simulink model "ThreePhaseBidirectional"  (R2020b)
settings: Solver=ode23t  StartTime=0.0  StopTime=0.5  RelTol=1e-3
libraries: powerlib x27, powerlib_meascontrol x6, pid_lib x4, eePowerMeasurement x4, simulink x2
settings Model: Creator=Matthew  LastModifiedBy=Matthew

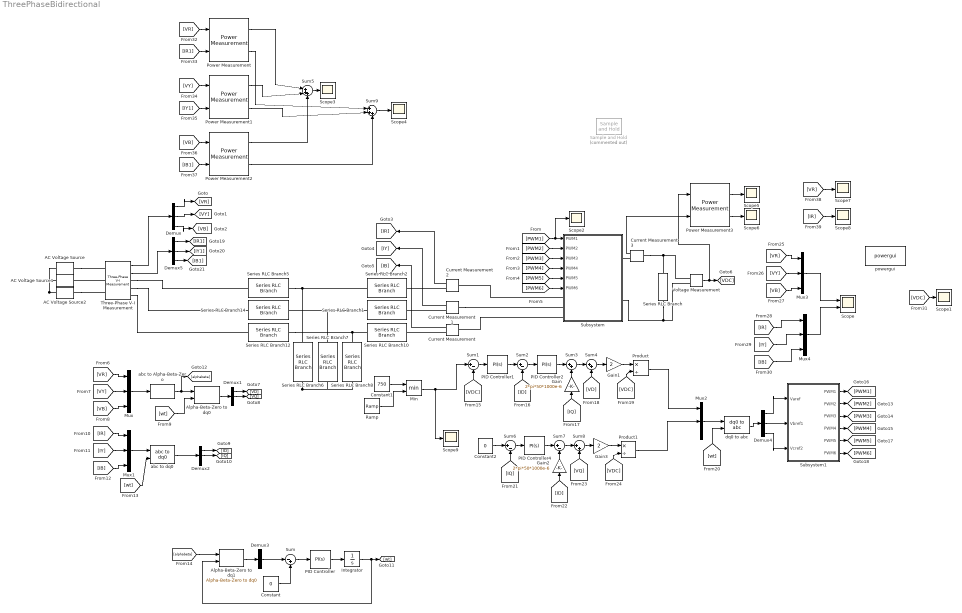
== system ThreePhaseBidirectional ==
  AC Voltage Source : powerlib/Electrical Sources/AC Voltage Source  Amplitude=350  Phase=0  Frequency=50  SampleTime=0  Measurements=None  BusType=swing  Pref=10e3  Qref=0  Qmin=-inf  Qmax=+inf
  AC Voltage Source1 : powerlib/Electrical Sources/AC Voltage Source  Amplitude=350  Phase=120  Frequency=50  SampleTime=0  Measurements=None  BusType=swing  Pref=10e3  Qref=0  Qmin=-inf  Qmax=+inf
  AC Voltage Source2 : powerlib/Electrical Sources/AC Voltage Source  Amplitude=350  Phase=240  Frequency=50  SampleTime=0  Measurements=None  BusType=swing  Pref=10e3  Qref=0  Qmin=-inf  Qmax=+inf
  Alpha-Beta-Zero to dq0 : powerlib_meascontrol/Transformations/Alpha-Beta-Zero to dq0  Alignment=90 degrees behind phase A axis
  Alpha-Beta-Zero to dq1 : powerlib_meascontrol/Transformations/Alpha-Beta-Zero to dq0  Alignment=90 degrees behind phase A axis
  Constant : Constant  Value=0
  Constant1 : Constant  Value=750
  Constant2 : Constant  Value=0
  Current Measurement{,1..3} (4 alike) : powerlib/Measurements/Current Measurement  PhasorSimulation=off  OutputType=Complex  PSBequivalent=0
  Demux{,1..5} (6 alike) : Demux  Outputs=3
  Gain : Gain  Gain=2*pi*50*1000e-6
  Gain1 : Gain  Gain=2
  Gain2 : Gain  Gain=2*pi*50*1000e-6
  Gain3 : Gain  Gain=2
  Integrator : Integrator
  Min : MinMax  Inputs=2
  Mux{,1..4} (5 alike) : Mux  Inputs=3
  PID Controller : pid_lib/PID Controller  Controller=PI  Form=Parallel  TimeDomain=Continuous-time  UseExternalTs=off  SampleTime=-1  IntegratorMethod=Forward Euler  FilterMethod=Forward Euler  ControllerParametersSource=internal  P=10  I=50000  D=0  UseFilter=on  N=100  TunerSelectOption=Transfer Function Based (PID Tuner App)  InitialConditionSource=internal  InitialConditionForIntegrator=0  InitialConditionForFilter=0  DifferentiatorICPrevScaledInput=0  ExternalReset=none  TrackingMode=off  Kt=1  LimitOutput=off  SatLimitsSource=internal  UpperSaturationLimit=inf  LowerSaturationLimit=-inf  LinearizeAsGain=on  AntiWindupMode=none  Kb=1  POutMin=[]  POutMax=[]  IOutMin=[]  IOutMax=[]  DOutMin=[]  DOutMax=[]  NOutMin=[]  NOutMax=[]  SumOutMin=[]  SumOutMax=[]  SaturationOutMin=[]  SaturationOutMax=[]  PParamMin=[]  PParamMax=[]  IParamMin=[]  IParamMax=[]  DParamMin=[]  DParamMax=[]  NParamMin=[]  NParamMax=[]  KbParamMin=[]  KbParamMax=[]  KtParamMin=[]  KtParamMax=[]  KbOutMin=[]  KbOutMax=[]  KtOutMin=[]  KtOutMax=[]  IntegratorOutMin=[]  IntegratorOutMax=[]  FilterOutMin=[]  FilterOutMax=[]  SumI1OutMin=[]  SumI1OutMax=[]  SumI2OutMin=[]  SumI2OutMax=[]  SumI3OutMin=[]  SumI3OutMax=[]  SumI4OutMin=[]  SumI4OutMax=[]  SumDOutMin=[]  SumDOutMax=[]  DifferentiatorOutMin=[]  DifferentiatorOutMax=[]  FilterDiffOutCoefMin=[]  FilterDiffOutCoefMax=[]  ReciprocalOutMin=[]  ReciprocalOutMax=[]  SumDenOutMin=[]  SumDenOutMax=[]  SumNumOutMin=[]  SumNumOutMax=[]  DivideOutMin=[]  DivideOutMax=[]  UdiffTsProdOutMin=[]  UdiffTsProdOutMax=[]  NTsProdOutMin=[]  NTsProdOutMax=[]  UintegralTsProdOutMin=[]  UintegralTsProdOutMax=[]  UngainTsProdOutMin=[]  UngainTsProdOutMax=[]  IntegratorContinuousStateAttributes=''  IntegratorStateMustResolveToSignalObject=off  IntegratorRTWStateStorageClass=Auto  FilterContinuousStateAttributes=''  FilterStateMustResolveToSignalObject=off  FilterRTWStateStorageClass=Auto  ParallelPVariant=InternalParameters  IdealPVariant=Disabled  IVariant=InternalParameters  DVariant=Disabled  IntegratorVariant=Continuous  SatVariant=Disabled  AWVariant=Passthrough  PCopyVariant=Disabled  TRVariant=Disabled  FdbkBlocksVariant=Forward  IdealPFdbkVariant=Disabled  SatFdbkVariant=Disabled  DerivativeFilterVariant=Disabled  NVariant=Disabled  NCopyVariant=Disabled_SignalSpec  FilterICVariant=Disabled  IntegratorICVariant=InternalICs  ExternalResetVariant=Disabled  TRSumVariant=Passthrough  SumFdbkVariant=Disabled  SumVariant=Sum_PI  TsampFilterVariant=InternalTs  TsampNgainVariant=Passthrough  TsampIntegralVariant=Passthrough  ExternalSaturationOutDataTypeStr=Inherit: Same as second input
  PID Controller1 : pid_lib/PID Controller  Controller=PI  Form=Parallel  TimeDomain=Continuous-time  UseExternalTs=off  SampleTime=-1  IntegratorMethod=Forward Euler  FilterMethod=Forward Euler  ControllerParametersSource=internal  P=0.5  I=200  D=0  UseFilter=on  N=100  TunerSelectOption=Transfer Function Based (PID Tuner App)  InitialConditionSource=internal  InitialConditionForIntegrator=0  InitialConditionForFilter=0  DifferentiatorICPrevScaledInput=0  ExternalReset=none  TrackingMode=off  Kt=1  LimitOutput=off  SatLimitsSource=internal  UpperSaturationLimit=inf  LowerSaturationLimit=-inf  LinearizeAsGain=on  AntiWindupMode=none  Kb=1  POutMin=[]  POutMax=[]  IOutMin=[]  IOutMax=[]  DOutMin=[]  DOutMax=[]  NOutMin=[]  NOutMax=[]  SumOutMin=[]  SumOutMax=[]  SaturationOutMin=[]  SaturationOutMax=[]  PParamMin=[]  PParamMax=[]  IParamMin=[]  IParamMax=[]  DParamMin=[]  DParamMax=[]  NParamMin=[]  NParamMax=[]  KbParamMin=[]  KbParamMax=[]  KtParamMin=[]  KtParamMax=[]  KbOutMin=[]  KbOutMax=[]  KtOutMin=[]  KtOutMax=[]  IntegratorOutMin=[]  IntegratorOutMax=[]  FilterOutMin=[]  FilterOutMax=[]  SumI1OutMin=[]  SumI1OutMax=[]  SumI2OutMin=[]  SumI2OutMax=[]  SumI3OutMin=[]  SumI3OutMax=[]  SumI4OutMin=[]  SumI4OutMax=[]  SumDOutMin=[]  SumDOutMax=[]  DifferentiatorOutMin=[]  DifferentiatorOutMax=[]  FilterDiffOutCoefMin=[]  FilterDiffOutCoefMax=[]  ReciprocalOutMin=[]  ReciprocalOutMax=[]  SumDenOutMin=[]  SumDenOutMax=[]  SumNumOutMin=[]  SumNumOutMax=[]  DivideOutMin=[]  DivideOutMax=[]  UdiffTsProdOutMin=[]  UdiffTsProdOutMax=[]  NTsProdOutMin=[]  NTsProdOutMax=[]  UintegralTsProdOutMin=[]  UintegralTsProdOutMax=[]  UngainTsProdOutMin=[]  UngainTsProdOutMax=[]  IntegratorContinuousStateAttributes=''  IntegratorStateMustResolveToSignalObject=off  IntegratorRTWStateStorageClass=Auto  FilterContinuousStateAttributes=''  FilterStateMustResolveToSignalObject=off  FilterRTWStateStorageClass=Auto  ParallelPVariant=InternalParameters  IdealPVariant=Disabled  IVariant=InternalParameters  DVariant=Disabled  IntegratorVariant=Continuous  SatVariant=Disabled  AWVariant=Passthrough  PCopyVariant=Disabled  TRVariant=Disabled  FdbkBlocksVariant=Forward  IdealPFdbkVariant=Disabled  SatFdbkVariant=Disabled  DerivativeFilterVariant=Disabled  NVariant=Disabled  NCopyVariant=Disabled_SignalSpec  FilterICVariant=Disabled  IntegratorICVariant=InternalICs  ExternalResetVariant=Disabled  TRSumVariant=Passthrough  SumFdbkVariant=Disabled  SumVariant=Sum_PI  TsampFilterVariant=InternalTs  TsampNgainVariant=Passthrough  TsampIntegralVariant=Passthrough  ExternalSaturationOutDataTypeStr=Inherit: Same as second input
  PID Controller2 : pid_lib/PID Controller  Controller=PI  Form=Parallel  TimeDomain=Continuous-time  UseExternalTs=off  SampleTime=-1  IntegratorMethod=Forward Euler  FilterMethod=Forward Euler  ControllerParametersSource=internal  P=25  I=500  D=0  UseFilter=on  N=100  TunerSelectOption=Transfer Function Based (PID Tuner App)  InitialConditionSource=internal  InitialConditionForIntegrator=0  InitialConditionForFilter=0  DifferentiatorICPrevScaledInput=0  ExternalReset=none  TrackingMode=off  Kt=1  LimitOutput=off  SatLimitsSource=internal  UpperSaturationLimit=inf  LowerSaturationLimit=-inf  LinearizeAsGain=on  AntiWindupMode=none  Kb=1  POutMin=[]  POutMax=[]  IOutMin=[]  IOutMax=[]  DOutMin=[]  DOutMax=[]  NOutMin=[]  NOutMax=[]  SumOutMin=[]  SumOutMax=[]  SaturationOutMin=[]  SaturationOutMax=[]  PParamMin=[]  PParamMax=[]  IParamMin=[]  IParamMax=[]  DParamMin=[]  DParamMax=[]  NParamMin=[]  NParamMax=[]  KbParamMin=[]  KbParamMax=[]  KtParamMin=[]  KtParamMax=[]  KbOutMin=[]  KbOutMax=[]  KtOutMin=[]  KtOutMax=[]  IntegratorOutMin=[]  IntegratorOutMax=[]  FilterOutMin=[]  FilterOutMax=[]  SumI1OutMin=[]  SumI1OutMax=[]  SumI2OutMin=[]  SumI2OutMax=[]  SumI3OutMin=[]  SumI3OutMax=[]  SumI4OutMin=[]  SumI4OutMax=[]  SumDOutMin=[]  SumDOutMax=[]  DifferentiatorOutMin=[]  DifferentiatorOutMax=[]  FilterDiffOutCoefMin=[]  FilterDiffOutCoefMax=[]  ReciprocalOutMin=[]  ReciprocalOutMax=[]  SumDenOutMin=[]  SumDenOutMax=[]  SumNumOutMin=[]  SumNumOutMax=[]  DivideOutMin=[]  DivideOutMax=[]  UdiffTsProdOutMin=[]  UdiffTsProdOutMax=[]  NTsProdOutMin=[]  NTsProdOutMax=[]  UintegralTsProdOutMin=[]  UintegralTsProdOutMax=[]  UngainTsProdOutMin=[]  UngainTsProdOutMax=[]  IntegratorContinuousStateAttributes=''  IntegratorStateMustResolveToSignalObject=off  IntegratorRTWStateStorageClass=Auto  FilterContinuousStateAttributes=''  FilterStateMustResolveToSignalObject=off  FilterRTWStateStorageClass=Auto  ParallelPVariant=InternalParameters  IdealPVariant=Disabled  IVariant=InternalParameters  DVariant=Disabled  IntegratorVariant=Continuous  SatVariant=Disabled  AWVariant=Passthrough  PCopyVariant=Disabled  TRVariant=Disabled  FdbkBlocksVariant=Forward  IdealPFdbkVariant=Disabled  SatFdbkVariant=Disabled  DerivativeFilterVariant=Disabled  NVariant=Disabled  NCopyVariant=Disabled_SignalSpec  FilterICVariant=Disabled  IntegratorICVariant=InternalICs  ExternalResetVariant=Disabled  TRSumVariant=Passthrough  SumFdbkVariant=Disabled  SumVariant=Sum_PI  TsampFilterVariant=InternalTs  TsampNgainVariant=Passthrough  TsampIntegralVariant=Passthrough  ExternalSaturationOutDataTypeStr=Inherit: Same as second input
  PID Controller4 : pid_lib/PID Controller  Controller=PI  Form=Parallel  TimeDomain=Continuous-time  UseExternalTs=off  SampleTime=-1  IntegratorMethod=Forward Euler  FilterMethod=Forward Euler  ControllerParametersSource=internal  P=25  I=500  D=0  UseFilter=on  N=100  TunerSelectOption=Transfer Function Based (PID Tuner App)  InitialConditionSource=internal  InitialConditionForIntegrator=0  InitialConditionForFilter=0  DifferentiatorICPrevScaledInput=0  ExternalReset=none  TrackingMode=off  Kt=1  LimitOutput=off  SatLimitsSource=internal  UpperSaturationLimit=inf  LowerSaturationLimit=-inf  LinearizeAsGain=on  AntiWindupMode=none  Kb=1  POutMin=[]  POutMax=[]  IOutMin=[]  IOutMax=[]  DOutMin=[]  DOutMax=[]  NOutMin=[]  NOutMax=[]  SumOutMin=[]  SumOutMax=[]  SaturationOutMin=[]  SaturationOutMax=[]  PParamMin=[]  PParamMax=[]  IParamMin=[]  IParamMax=[]  DParamMin=[]  DParamMax=[]  NParamMin=[]  NParamMax=[]  KbParamMin=[]  KbParamMax=[]  KtParamMin=[]  KtParamMax=[]  KbOutMin=[]  KbOutMax=[]  KtOutMin=[]  KtOutMax=[]  IntegratorOutMin=[]  IntegratorOutMax=[]  FilterOutMin=[]  FilterOutMax=[]  SumI1OutMin=[]  SumI1OutMax=[]  SumI2OutMin=[]  SumI2OutMax=[]  SumI3OutMin=[]  SumI3OutMax=[]  SumI4OutMin=[]  SumI4OutMax=[]  SumDOutMin=[]  SumDOutMax=[]  DifferentiatorOutMin=[]  DifferentiatorOutMax=[]  FilterDiffOutCoefMin=[]  FilterDiffOutCoefMax=[]  ReciprocalOutMin=[]  ReciprocalOutMax=[]  SumDenOutMin=[]  SumDenOutMax=[]  SumNumOutMin=[]  SumNumOutMax=[]  DivideOutMin=[]  DivideOutMax=[]  UdiffTsProdOutMin=[]  UdiffTsProdOutMax=[]  NTsProdOutMin=[]  NTsProdOutMax=[]  UintegralTsProdOutMin=[]  UintegralTsProdOutMax=[]  UngainTsProdOutMin=[]  UngainTsProdOutMax=[]  IntegratorContinuousStateAttributes=''  IntegratorStateMustResolveToSignalObject=off  IntegratorRTWStateStorageClass=Auto  FilterContinuousStateAttributes=''  FilterStateMustResolveToSignalObject=off  FilterRTWStateStorageClass=Auto  ParallelPVariant=InternalParameters  IdealPVariant=Disabled  IVariant=InternalParameters  DVariant=Disabled  IntegratorVariant=Continuous  SatVariant=Disabled  AWVariant=Passthrough  PCopyVariant=Disabled  TRVariant=Disabled  FdbkBlocksVariant=Forward  IdealPFdbkVariant=Disabled  SatFdbkVariant=Disabled  DerivativeFilterVariant=Disabled  NVariant=Disabled  NCopyVariant=Disabled_SignalSpec  FilterICVariant=Disabled  IntegratorICVariant=InternalICs  ExternalResetVariant=Disabled  TRSumVariant=Passthrough  SumFdbkVariant=Disabled  SumVariant=Sum_PI  TsampFilterVariant=InternalTs  TsampNgainVariant=Passthrough  TsampIntegralVariant=Passthrough  ExternalSaturationOutDataTypeStr=Inherit: Same as second input
  Power Measurement : eePowerMeasurement/Power Measurement  LabelModeActiveChoice=Continuous  F=50  K=[1]  Ts=0
      settings: SourceProductBaseCode=PS
  Power Measurement1 : eePowerMeasurement/Power Measurement  LabelModeActiveChoice=Continuous  F=50  K=[1]  Ts=0
      settings: SourceProductBaseCode=PS
  Power Measurement2 : eePowerMeasurement/Power Measurement  LabelModeActiveChoice=Continuous  F=50  K=[1]  Ts=0
      settings: SourceProductBaseCode=PS
  Power Measurement3 : eePowerMeasurement/Power Measurement  LabelModeActiveChoice=Continuous  F=50  K=[0 1]  Ts=0
      settings: SourceProductBaseCode=PS
  Product : Product  Inputs=*/
  Product1 : Product  Inputs=*/
  Ramp : simulink/Sources/Ramp  slope=1136  start=0  InitialOutput=608
  Sample and Hold : powerlib_meascontrol/Additional Components/Sample and Hold  Commented=on  ic=0  Ts=0
      settings: SourceProductBaseCode=PS
  Scope : Scope  NumInputPorts=2
  Scope{1..9} (9 alike) : Scope
  Series RLC Branch : powerlib/Elements/Series RLC Branch  LConnTagsString=__new0  RConnTagsString=__new0  BranchType=R  Resistance=6.4  Inductance=1e-3  SetiL0=off  InitialCurrent=0  Capacitance=1e-6  Setx0=off  InitialVoltage=0  Measurements=None
  Series RLC Branch{1..2,5,10,12,14} (6 alike) : powerlib/Elements/Series RLC Branch  LConnTagsString=__new0  RConnTagsString=__new0  BranchType=L  Resistance=1  Inductance=500e-6  SetiL0=off  InitialCurrent=0  Capacitance=0  Setx0=off  InitialVoltage=0  Measurements=None
  Series RLC Branch6 : powerlib/Elements/Series RLC Branch  LConnTagsString=__new0  RConnTagsString=__new0  BranchType=C  Resistance=1  Inductance=1e-3  SetiL0=off  InitialCurrent=0  Capacitance=100e-6  Setx0=off  InitialVoltage=0  Measurements=None
  Series RLC Branch7 : powerlib/Elements/Series RLC Branch  LConnTagsString=__new0  RConnTagsString=__new0  BranchType=C  Resistance=1  Inductance=1e-3  SetiL0=off  InitialCurrent=0  Capacitance=100e-6  Setx0=off  InitialVoltage=0  Measurements=None
  Series RLC Branch8 : powerlib/Elements/Series RLC Branch  LConnTagsString=__new0  RConnTagsString=__new0  BranchType=C  Resistance=1  Inductance=1e-3  SetiL0=off  InitialCurrent=0  Capacitance=100e-6  Setx0=off  InitialVoltage=0  Measurements=None
  Subsystem : Subsystem
  Subsystem1 : Subsystem
  Sum : Sum  Inputs=|-+
  Sum{1..2,6..7} (4 alike) : Sum  Inputs=|+-
  Sum3 : Sum  Inputs=|++
  Sum4 : Sum  Inputs=|++
  Sum5 : Sum  Inputs=|+++
  Sum8 : Sum  Inputs=|++
  Sum9 : Sum  Inputs=|+++
  Three-Phase V-I Measurement : powerlib/Measurements/Three-Phase V-I Measurement  VoltageMeasurement=phase-to-phase  SetLabelV=off  LabelV=Vabc  Vpu=off  VpuLL=off  CurrentMeasurement=yes  SetLabelI=off  LabelI=Iabc  Ipu=off  Pbase=100e6  Vbase=500e3  OutputType=Complex  PhasorSimulation=off  PSBequivalent=0
  Voltage Measurement : powerlib/Measurements/Voltage Measurement  PhasorSimulation=off  OutputType=Complex  PSBequivalent=0
  abc to Alpha-Beta-Zero : powerlib_meascontrol/Transformations/abc to Alpha-Beta-Zero
  abc to dq0 : powerlib_meascontrol/Transformations/abc to dq0  Alignment=90 degrees behind phase A axis
  dq0 to abc : powerlib_meascontrol/Transformations/dq0 to abc  Alignment=90 degrees behind phase A axis
  powergui : powerlib/powergui  Priority=1  SimulationMode=Discrete  SampleTime=1e-6  frequency=60  Iterations=50  frequencyindice=50  Pbase=100e6  ErrMax=1e-4  UnitsV=kV  UnitsW=MW  buscounter=0  FunctionMessages=off  echomessages=off  EnableUseOfTLC=off  CurrentSourceSwitches=off  DisableSnubberDevices=off  DisableRonSwitches=off  DisableVfSwitches=off  DisplayEquations=off  AutomaticDiscreteSolvers=off  SolverType=Tustin/Backward Euler (TBE)  Interpol=off  ExternalGateDelay=off  methode=off  Ts=100  x0status=blocks  SPID=on  SwTol=0  HookPort=off  NonlinearTolerance=1e-4  nMaxIteration=100  ContinueOnMaxIteration=off  RestoreLinks=warning  ResistiveCurrentMeasurement=off  Frange=[0:2:500]  Ylog=off  Xlog=on  ShowGrid=off  save=off  variable=ZData  structure=0  ZoomFFT=off  StartTime=0.0  cycles=1  DisplayStyle=1  fundamental=60  FreqAxis=off  MaxFrequency=1000  frequencyindicesteady=1  RmsSteady=1  display=off
  wires:
  Three-Phase V-I Measurement/1 -> Demux/1
  Demux/1 -> [VR]
  Demux/2 -> [VY]
  Demux/3 -> [VB]
  Current Measurement2/1 -> [IR]
  Current Measurement1/1 -> [IY]
  Current Measurement/1 -> [IB]
  [PWM1] -> Scope2/1, Subsystem/1(PWM1)
  [PWM2] -> Subsystem/2(PWM2)
  [PWM3] -> Subsystem/3(PWM3)
  [PWM4] -> Subsystem/4(PWM4)
  [PWM5] -> Subsystem/5(PWM5)
  [PWM6] -> Subsystem/6(PWM6)
  Voltage Measurement/1 -> Power Measurement3/1, [VDC]
  [VR] -> Mux/1
  [VB] -> Mux/3
  [VY] -> Mux/2
  Mux/1 -> abc to Alpha-Beta-Zero/1
  abc to Alpha-Beta-Zero/1 -> [alphabeta], Alpha-Beta-Zero to dq0/1
  [wt] -> Alpha-Beta-Zero to dq0/2
  Alpha-Beta-Zero to dq0/1 -> Demux1/1
  Demux1/1 -> [VD]
  Demux1/2 -> [VQ]
  Demux2/2 -> [IQ]
  Demux2/1 -> [ID]
  abc to dq0/1 -> Demux2/1
  Mux1/1 -> abc to dq0/1
  [IY] -> Mux1/2
  [IB] -> Mux1/3
  [IR] -> Mux1/1
  [wt] -> abc to dq0/2
  Alpha-Beta-Zero to dq1/1 -> Demux3/1
  Demux3/2 -> Sum/1
  Constant/1 -> Sum/2
  Sum/1 -> PID Controller/1
  PID Controller/1 -> Integrator/1
  Integrator/1 -> [wt], Alpha-Beta-Zero to dq1/2
  [alphabeta] -> Alpha-Beta-Zero to dq1/1
  [VDC] -> Sum1/2
  Sum1/1 -> PID Controller1/1
  PID Controller1/1 -> Sum2/1
  [ID] -> Sum2/2
  Sum2/1 -> PID Controller2/1
  Gain/1 -> Sum3/2
  PID Controller2/1 -> Sum3/1
  [IQ] -> Gain/1
  Sum3/1 -> Sum4/1
  [VD] -> Sum4/2
  Sum4/1 -> Gain1/1
  Gain1/1 -> Product/1
  [VDC] -> Product/2
  Product/1 -> Mux2/1
  [VDC] -> Product1/2
  Gain3/1 -> Product1/1
  Sum8/1 -> Gain3/1
  [VQ] -> Sum8/2
  Sum7/1 -> Sum8/1
  [ID] -> Gain2/1
  PID Controller4/1 -> Sum7/1
  Gain2/1 -> Sum7/2
  Sum6/1 -> PID Controller4/1
  [IQ] -> Sum6/2
  Constant2/1 -> Sum6/1
  Product1/1 -> Mux2/2
  Mux2/1 -> dq0 to abc/1
  [wt] -> dq0 to abc/2
  dq0 to abc/1 -> Demux4/1
  Demux4/1 -> Subsystem1/1(Varef)
  Demux4/2 -> Subsystem1/2(Vbref1)
  Demux4/3 -> Subsystem1/3(Vcref2)
  Subsystem1/1(PWM1) -> [PWM1]
  Subsystem1/2(PWM2) -> [PWM2]
  Subsystem1/3(PWM3) -> [PWM3]
  Subsystem1/4(PWM4) -> [PWM4]
  Subsystem1/5(PWM5) -> [PWM5]
  Subsystem1/6(PWM6) -> [PWM6]
  [VR] -> Mux3/1
  [VY] -> Mux3/2
  Mux3/1 -> Scope/1
  [VB] -> Mux3/3
  Mux4/1 -> Scope/2
  [IY] -> Mux4/2
  [IB] -> Mux4/3
  [IR] -> Mux4/1
  [VDC] -> Scope1/1
  [VR] -> Power Measurement/1
  [IR1] -> Power Measurement/2
  Power Measurement/1 -> Sum5/1
  Power Measurement/2 -> Sum9/1
  [VY] -> Power Measurement1/1
  [IY1] -> Power Measurement1/2
  [VB] -> Power Measurement2/1
  [IB1] -> Power Measurement2/2
  Power Measurement1/1 -> Sum5/2
  Power Measurement2/1 -> Sum5/3
  Sum5/1 -> Scope3/1
  Power Measurement1/2 -> Sum9/2
  Power Measurement2/2 -> Sum9/3
  Sum9/1 -> Scope4/1
  Current Measurement3/1 -> Power Measurement3/2
  Power Measurement3/1 -> Scope5/1
  Power Measurement3/2 -> Scope6/1
  Demux5/1 -> [IR1]
  Three-Phase V-I Measurement/2 -> Demux5/1
  Demux5/3 -> [IB1]
  Demux5/2 -> [IY1]
  [VR] -> Scope7/1
  [IR] -> Scope8/1
  Ramp/1 -> Min/2
  Min/1 -> Scope9/1, Sum1/1
  Constant1/1 -> Min/1
  connections:
  Series RLC Branch7/LConn1 -- Series RLC Branch1/RConn1 -- Series RLC Branch14/LConn1
  Series RLC Branch6/LConn1 -- Series RLC Branch5/LConn1 -- Series RLC Branch2/RConn1
  AC Voltage Source2/LConn1 -- AC Voltage Source/LConn1 -- AC Voltage Source1/LConn1
  Series RLC Branch6/RConn1 -- Series RLC Branch8/RConn1 -- Series RLC Branch7/RConn1
  Series RLC Branch10/RConn1 -- Series RLC Branch12/LConn1 -- Series RLC Branch8/LConn1
  AC Voltage Source2/RConn1 -- Three-Phase V-I Measurement/LConn3
  Three-Phase V-I Measurement/LConn2 -- AC Voltage Source1/RConn1
  AC Voltage Source/RConn1 -- Three-Phase V-I Measurement/LConn1
  Three-Phase V-I Measurement/RConn1 -- Series RLC Branch5/RConn1
  Three-Phase V-I Measurement/RConn2 -- Series RLC Branch14/RConn1
  Three-Phase V-I Measurement/RConn3 -- Series RLC Branch12/RConn1
  Current Measurement/RConn1 -- Series RLC Branch10/LConn1
  Current Measurement2/RConn1 -- Series RLC Branch2/LConn1
  Current Measurement1/RConn1 -- Series RLC Branch1/LConn1
  Current Measurement1/LConn1 -- Subsystem/LConn2
  Subsystem/LConn3 -- Current Measurement/LConn1
  Subsystem/LConn1 -- Current Measurement2/LConn1
  Series RLC Branch/LConn1 -- Current Measurement3/LConn1 -- Voltage Measurement/LConn1
  Current Measurement3/RConn1 -- Subsystem/RConn1
  Subsystem/RConn2 -- Series RLC Branch/RConn1 -- Voltage Measurement/LConn2

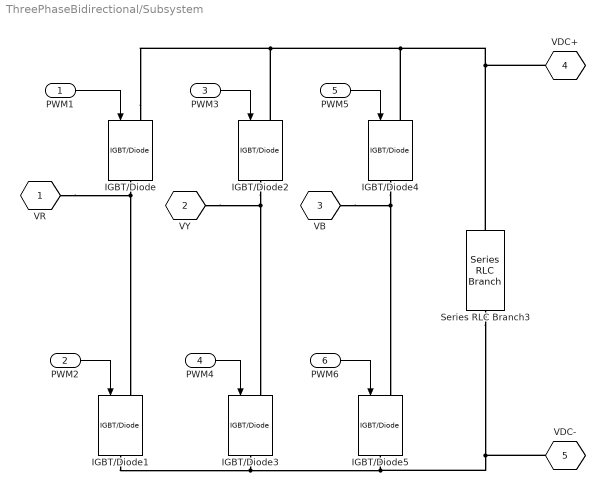
== system ThreePhaseBidirectional/Subsystem ==
  PWM1 : Inport
  PWM2 : Inport  Port=2
  PWM3 : Inport  Port=3
  PWM4 : Inport  Port=4
  PWM5 : Inport  Port=5
  PWM6 : Inport  Port=6
  IGBT/Diode{,1..5} (6 alike) : powerlib/Power Electronics/IGBT//Diode  Ron=1e-3  Rs=1e5  Cs=inf  Measurements=off
  Series RLC Branch3 : powerlib/Elements/Series RLC Branch  LConnTagsString=__new0  RConnTagsString=__new0  BranchType=RC  Resistance=1e-3  Inductance=1e-3  SetiL0=off  InitialCurrent=0  Capacitance=5600e-6  Setx0=off  InitialVoltage=0  Measurements=None
  VR : PMIOPort  Tag=PMCPort  Side=Left
  VY : PMIOPort  Tag=PMCPort  Port=2  Side=Left
  VB : PMIOPort  Tag=PMCPort  Port=3  Side=Left
  VDC+ : PMIOPort  Tag=PMCPort  Port=4  Side=Right
  VDC- : PMIOPort  Tag=PMCPort  Port=5  Side=Right
  wires:
  PWM2/1 -> IGBT/Diode1/1
  PWM3/1 -> IGBT/Diode2/1
  PWM4/1 -> IGBT/Diode3/1
  PWM6/1 -> IGBT/Diode5/1
  PWM5/1 -> IGBT/Diode4/1
  PWM1/1 -> IGBT/Diode/1
  connections:
  IGBT/Diode/LConn1 -- VDC+/RConn1 -- Series RLC Branch3/LConn1 -- IGBT/Diode4/LConn1 -- IGBT/Diode2/LConn1
  IGBT/Diode4/RConn1 -- VB/RConn1 -- IGBT/Diode5/LConn1
  IGBT/Diode5/RConn1 -- VDC-/RConn1 -- Series RLC Branch3/RConn1 -- IGBT/Diode3/RConn1 -- IGBT/Diode1/RConn1
  IGBT/Diode2/RConn1 -- VY/RConn1 -- IGBT/Diode3/LConn1
  IGBT/Diode/RConn1 -- VR/RConn1 -- IGBT/Diode1/LConn1

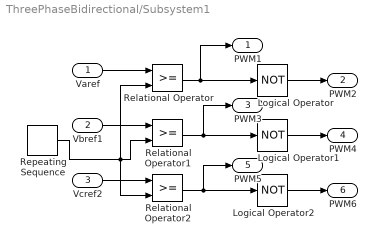
== system ThreePhaseBidirectional/Subsystem1 ==
  Varef : Inport
  Vbref1 : Inport  Port=2
  Vcref2 : Inport  Port=3
  Logical Operator : Logic  Operator=NOT  AllPortsSameDT=off  OutDataTypeStr=boolean
  Logical Operator1 : Logic  Operator=NOT  AllPortsSameDT=off  OutDataTypeStr=boolean
  Logical Operator2 : Logic  Operator=NOT  AllPortsSameDT=off  OutDataTypeStr=boolean
  Relational Operator : RelationalOperator  OutDataTypeStr=boolean  RndMeth=Simplest
  Relational Operator1 : RelationalOperator  OutDataTypeStr=boolean  RndMeth=Simplest
  Relational Operator2 : RelationalOperator  OutDataTypeStr=boolean  RndMeth=Simplest
  Repeating Sequence : simulink/Sources/Repeating Sequence  rep_seq_t=[0 0.00005 0.0001]  rep_seq_y=[-1 1 -1]
  PWM1 : Outport
  PWM2 : Outport  Port=2
  PWM3 : Outport  Port=3
  PWM4 : Outport  Port=4
  PWM5 : Outport  Port=5
  PWM6 : Outport  Port=6
  wires:
  Logical Operator2/1 -> PWM6/1
  Relational Operator2/1 -> PWM5/1, Logical Operator2/1
  Vcref2/1 -> Relational Operator2/1
  Vbref1/1 -> Relational Operator1/1
  Logical Operator/1 -> PWM2/1
  Repeating Sequence/1 -> Relational Operator2/2, Relational Operator/2, Relational Operator1/2
  Relational Operator1/1 -> PWM3/1, Logical Operator1/1
  Relational Operator/1 -> PWM1/1, Logical Operator/1
  Logical Operator1/1 -> PWM4/1
  Varef/1 -> Relational Operator/1
